simulink model "template"  (R2021a)
settings: Solver=ode1  StartTime=0.0  StopTime=120  FixedStep=0.001  RelTol=1e-3
undefined symbols (not defined in the file or in its folder): Serial_Port, Standard_Devices
libraries: sldrtlib x2
settings Model: Creator=Mesih  LastModifiedBy=Mesih
settings SolverCC: AlgebraicLoopSolver=TrustRegion
settings DebuggingCC: SFMachineParentedDataDiag=warning
settings RTWCC: Description=Simulink Desktop Real-Time  SystemTargetFile=sldrt.tlc  TemplateMakefile=sldrt.tmf  RTWCompilerOptimization=on
settings CodeAppCC: MaxIdLength=95
settings SimulinkDesktopRealTimeCC: TargetPreCompLibLocation=C:\Program Files\Polyspace\R2021a\toolbox\sldrt\lib\win64

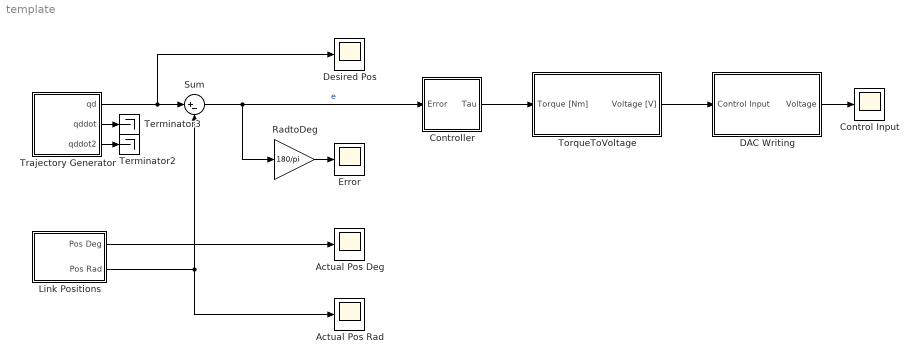
== system template ==
  Actual Pos Deg : Scope
  Actual Pos Rad : Scope
  Control Input : Scope
  Controller : Subsystem
  DAC Writing : Subsystem
  Desired Pos : Scope
  Error : Scope
  Link Positions : Subsystem
  RadtoDeg : Gain  Gain=180/pi
  Sum : Sum  Inputs=|+-
  Terminator2 : Terminator
  Terminator3 : Terminator
  TorqueToVoltage : Subsystem
  Trajectory Generator : Subsystem  mask{ampl=[0.6 0.7 0.4], freq=[1.0 1.0 1.0]}
      mask prompts: ampl "Amplitute"; freq "Frequency"
  wires:
  Trajectory Generator/1(qd) -> Desired Pos/1, Sum/1
  Link Positions/2(Pos Rad) -> Sum/2, Actual Pos Rad/1
  Link Positions/1(Pos Deg) -> Actual Pos Deg/1
  Sum/1 -> Controller/1(Error), RadtoDeg/1  "e"
  DAC Writing/1(Voltage) -> Control Input/1
  RadtoDeg/1 -> Error/1
  Trajectory Generator/3(qddot2) -> Terminator2/1
  Trajectory Generator/2(qddot) -> Terminator3/1
  TorqueToVoltage/1(Voltage [V]) -> DAC Writing/1(Control Input)
  Controller/1(Tau) -> TorqueToVoltage/1(Torque [Nm])

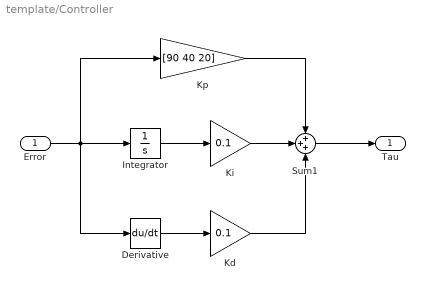
== system template/Controller ==
  Error : Inport
  Derivative : Derivative
  Integrator : Integrator
  Kd : Gain  Gain=0.1
  Ki : Gain  Gain=0.1
  Kp : Gain  Gain=[90 40 20]
  Sum1 : Sum  Inputs=+++
  Tau : Outport
  wires:
  Sum1/1 -> Tau/1
  Derivative/1 -> Kd/1
  Error/1 -> Integrator/1, Kp/1, Derivative/1
  Integrator/1 -> Ki/1
  Kp/1 -> Sum1/1
  Kd/1 -> Sum1/3
  Ki/1 -> Sum1/2

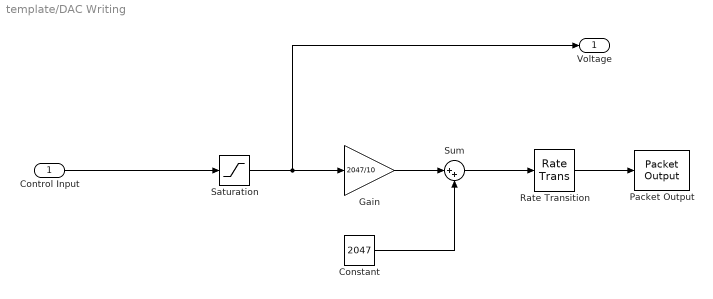
== system template/DAC Writing ==
  Control Input : Inport
  Constant : Constant  Value=2047
  Gain : Gain  Gain=2047/10
  Packet Output : sldrtlib/Packet Output  SampleTime=-1  MaxMissedTicks=1  ShowMissedTicks=off  YieldWhenWaiting=on  DrvName=Standard_Devices/Serial_Port  DrvAddress=6  DrvOptions=[256000 8 0 0 0 0 0 0]  PacketSize=6  DataTypes='3*uint16'  ShowReady=off  ShowError=off  PacketID=1  ByteOrder=1  InitialValue=[]  FinalValue=[]
      settings: AttributesFormatString=Serial Port [6]
  Rate Transition : RateTransition  Deterministic=off  OutPortSampleTimeOpt=Inherit
  Saturation : Saturate  UpperLimit=[10 10 10]  LowerLimit=[-10 -10 -10]
  Sum : Sum  Inputs=|++
  Voltage : Outport
  wires:
  Rate Transition/1 -> Packet Output/1
  Saturation/1 -> Voltage/1, Gain/1
  Gain/1 -> Sum/1
  Sum/1 -> Rate Transition/1
  Constant/1 -> Sum/2
  Control Input/1 -> Saturation/1

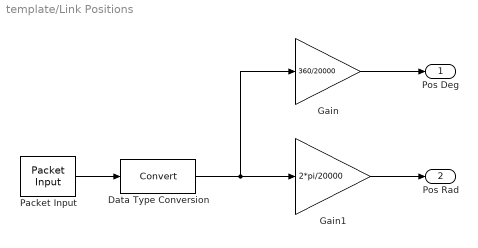
== system template/Link Positions ==
  Data Type Conversion : DataTypeConversion
  Gain : Gain  Gain=360/20000
  Gain1 : Gain  Gain=2*pi/20000
  Packet Input : sldrtlib/Packet Input  SampleTime=-1  MaxMissedTicks=1  ShowMissedTicks=off  YieldWhenWaiting=on  DrvName=Standard_Devices/Serial_Port  DrvAddress=6  DrvOptions=[256000 8 0 0 0 0 0 0]  PacketSize=6  DataTypes='3*int16'  ShowReady=off  ShowError=off  PacketID=1  ByteOrder=1  ShowTimestamp=off
      settings: AttributesFormatString=Serial Port [6]
  Pos Deg : Outport
  Pos Rad : Outport  Port=2
  wires:
  Data Type Conversion/1 -> Gain1/1, Gain/1
  Gain/1 -> Pos Deg/1
  Packet Input/1 -> Data Type Conversion/1
  Gain1/1 -> Pos Rad/1

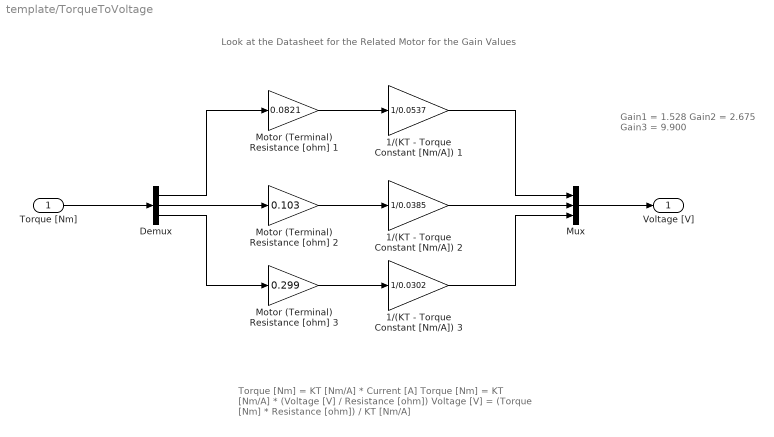
== system template/TorqueToVoltage ==
  note: Gain1 = 1.528
      | Gain2 = 2.675
      | Gain3 = 9.900
  note: Look at the Datasheet for the Related Motor for the Gain Values
  note: Torque [Nm] = KT [Nm/A] * Current [A]
      | Torque [Nm] = KT [Nm/A] * (Voltage [V] / Resistance [ohm])
      |
      | Voltage [V] = (Torque [Nm] * Resistance [ohm]) / KT [Nm/A]
  Torque [Nm] : Inport
  1/(KT - Torque Constant [Nm/A]) 1 : Gain  Gain=1/0.0537
  1/(KT - Torque Constant [Nm/A]) 2 : Gain  Gain=1/0.0385
  "1/(KT - Torque Constant [Nm/A]) 3 " : Gain  Gain=1/0.0302
  Demux : Demux  Outputs=3
  Motor (Terminal) Resistance [ohm] 1 : Gain  Gain=0.0821
  Motor (Terminal) Resistance [ohm] 2 : Gain  Gain=0.103
  Motor (Terminal) Resistance [ohm] 3 : Gain  Gain=0.299
  Mux : Mux  Inputs=3
  Voltage [V] : Outport
  wires:
  Motor (Terminal) Resistance [ohm] 3/1 -> "1/(KT - Torque Constant [Nm/A]) 3 "/1
  Motor (Terminal) Resistance [ohm] 2/1 -> 1/(KT - Torque Constant [Nm/A]) 2/1
  Motor (Terminal) Resistance [ohm] 1/1 -> 1/(KT - Torque Constant [Nm/A]) 1/1
  Torque [Nm]/1 -> Demux/1
  Demux/2 -> Motor (Terminal) Resistance [ohm] 2/1
  Demux/1 -> Motor (Terminal) Resistance [ohm] 1/1
  Demux/3 -> Motor (Terminal) Resistance [ohm] 3/1
  1/(KT - Torque Constant [Nm/A]) 2/1 -> Mux/2
  1/(KT - Torque Constant [Nm/A]) 1/1 -> Mux/1
  "1/(KT - Torque Constant [Nm/A]) 3 "/1 -> Mux/3
  Mux/1 -> Voltage [V]/1

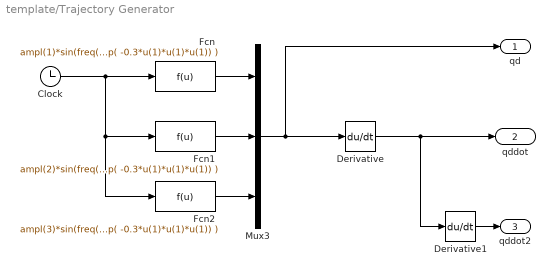
== system template/Trajectory Generator ==
  Clock : Clock
  Derivative : Derivative
  Derivative1 : Derivative
  Fcn : Fcn  Expr=ampl(1)*sin(freq(1)*u(1))*( 1-exp( -0.3*u(1)*u(1)*u(1)) )
  Fcn1 : Fcn  Expr=ampl(2)*sin(freq(2)*u(1))*( 1-exp( -0.3*u(1)*u(1)*u(1)) )
  Fcn2 : Fcn  Expr=ampl(3)*sin(freq(3)*u(1))*( 1-exp( -0.3*u(1)*u(1)*u(1)) )
  Mux3 : Mux  Inputs=3
  qd : Outport  VectorParamsAs1DForOutWhenUnconnected=off
  qddot : Outport  Port=2  VectorParamsAs1DForOutWhenUnconnected=off
  qddot2 : Outport  Port=3  VectorParamsAs1DForOutWhenUnconnected=off
  wires:
  Clock/1 -> Fcn/1, Fcn2/1, Fcn1/1
  Fcn/1 -> Mux3/1
  Fcn1/1 -> Mux3/2
  Mux3/1 -> qd/1, Derivative/1
  Derivative/1 -> qddot/1, Derivative1/1
  Derivative1/1 -> qddot2/1
  Fcn2/1 -> Mux3/3
